simulink model "Two_cars_multi_agent"  (Simulink 8.3)
settings: Solver=ode45  StartTime=0  StopTime=5  FixedStep=0.1  RelTol=1e-3
PreLoadFcn:
  | d1 = density.Data(2:end);
  | d1 = d1(2:end);
  | mean(d1)
libraries: simulink_extras x9, Solver_SF x3, truetime x3
settings Model: Creator=dhall  LastModifiedBy=Ye  SimulationMode=accelerator  ExtModeTrigMode=oneshot  ExtModeArmWhenConnect=off
settings DataIOCC: LimitDataPoints=off  SignalLoggingName=sigsOut
settings OptimizationCC: BooleanDataType=off  LocalBlockOutputs=off  InitFltsAndDblsToZero=on
settings DebuggingCC: ReadBeforeWriteMsg=DisableAll  WriteAfterWriteMsg=DisableAll  WriteAfterReadMsg=DisableAll  SaveWithParameterizedLinksMsg=none  SolverPrmCheckMsg=none  MultiTaskDSMMsg=none  MultiTaskCondExecSysMsg=none  StateNameClashWarn=none
settings HardwareCC: TargetIntDivRoundTo=Zero  TargetEndianess=LittleEndian  TargetHWDeviceType=MATLAB Host  ProdEqTarget=off
settings ModelReferenceCC: UpdateModelReferenceTargets=IfOutOfDate
settings SFSimCC: SFSimEnableDebug=off  SFSimOverflowDetection=off  SFSimEcho=off
settings RTWCC: IncludeERTFirstTime=on
settings GRTTargetCC: TargetFcnLib=ansi_tfl_tmw.mat  CompOptLevelCompliant=off

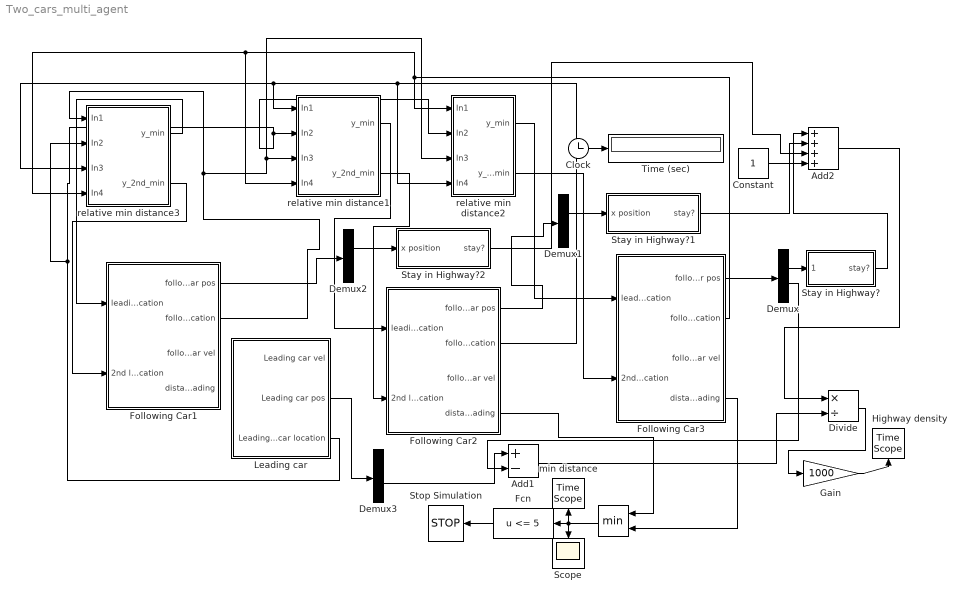
== system Two_cars_multi_agent ==
  " " : MinMax  Inputs=2  SampleTime=0.1
  Add1 : Sum  Inputs=+-
  Add2 : Sum  Inputs=++++
  Clock : Clock
  Constant : Constant
  Demux{,1..3} (4 alike) : Demux
  Divide : Product  Inputs=*/  RndMeth=Ceiling
  Fcn : Fcn  Expr=u <= 5
  "Following Car1 " : Subsystem
  Following Car2 : Subsystem
  Following Car3 : Subsystem
  Gain : Gain  Gain=1000
  Highway density : TimeScope  DefaultConfigurationName=spbscopes.TimeScopeBlockCfg  ScopeSpecification=DataTag1
  Leading car : Subsystem
  Scope : Scope
      settings: YMin=0  YMax=50  SaveName=ScopeData2
  Stay in Highway? : Subsystem
  Stay in Highway?1 : Subsystem
  Stay in Highway?2 : Subsystem
  Stop Simulation : Stop
  Time (sec) : Display
      settings: Format=bank  Decimation=100
  min distance : TimeScope  DefaultConfigurationName=spbscopes.TimeScopeBlockCfg  ScopeSpecification=DataTag2
  relative min distance1 : Subsystem
  relative min distance2 : Subsystem
  relative min distance3 : Subsystem
  wires:
  Clock/1 -> Time (sec)/1
  Fcn/1 -> Stop Simulation/1
  "Following Car1 "/2(following car location) -> relative min distance1/3(In3), relative min distance2/3(In3), relative min distance3/1(In1)
  Leading car/3(Leading car location) -> relative min distance2/2(In2), relative min distance1/2(In2), relative min distance3/2(In2)
  Leading car/2(Leading car pos) -> Demux3/1
  Following Car2/1(following car pos) -> Demux1/1
  Following Car2/2(following car location) -> relative min distance2/4(In4), relative min distance3/3(In3), relative min distance1/1(In1)
  Following Car3/1(following car pos) -> Demux/1
  Following Car3/2(following car location) -> relative min distance3/4(In4), relative min distance1/4(In4), relative min distance2/1(In1)
  relative min distance3/1(y_min) -> "Following Car1 "/1(leading car location)
  relative min distance1/1(y_min) -> Following Car2/1(leading car location)
  relative min distance2/1(y_min) -> Following Car3/1(leading car location)
  Add1/1 -> Divide/2
  Demux/2 -> Stay in Highway?/1(x position)
  Stay in Highway?/1(stay?) -> Add2/1
  Demux1/2 -> Stay in Highway?1/1(x position)
  Stay in Highway?1/1(stay?) -> Add2/2
  Demux2/2 -> Stay in Highway?2/1(x position)
  Stay in Highway?2/1(stay?) -> Add2/3
  Demux3/3 -> Add1/1
  Demux/3 -> Add1/2
  Constant/1 -> Add2/4
  Divide/1 -> Gain/1
  Add2/1 -> Divide/1
  Gain/1 -> Highway density/1
  relative min distance2/2(y_2nd_min) -> Following Car3/2(2nd leading car location)
  "Following Car1 "/1(following car pos) -> Demux2/1
  relative min distance1/2(y_2nd_min) -> Following Car2/2(2nd leading car location)
  relative min distance3/2(y_2nd_min) -> "Following Car1 "/2(2nd leading car location)
  Following Car2/4(distance leading) -> " "/1
  " "/1 -> Scope/1, Fcn/1, min distance/1
  Following Car3/4(distance leading) -> " "/2

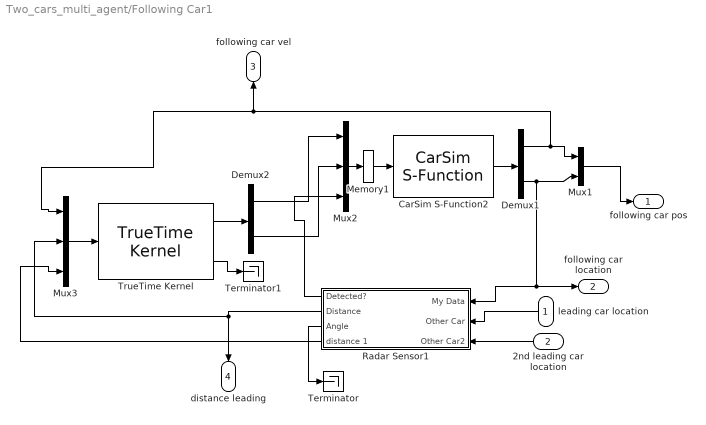
== system Two_cars_multi_agent/Following Car1  ==
  leading car location : Inport
  2nd leading car location : Inport  Port=2
  CarSim S-Function2 : Solver_SF/CarSim S-Function  Priority=1  VehicleCode=i_i2  SIMFILE=following_car_1.sim
  Demux1 : Demux  Outputs=[1 3]
  Demux2 : Demux  Outputs=[1 1]
  Memory1 : Memory
  Mux1 : Mux  Inputs=2
  Mux2 : Mux  Inputs=3
  Mux3 : Mux  Inputs=3
  Radar Sensor1 : Subsystem  mask{S_ANGLE=360, S_DISTANCE=700}
      mask prompts: S_ANGLE "View Angle (deg)"; S_DISTANCE "Distance Range (m)"
      mask help:
      | An example of a radar sensor. It can detect the distance between the sensor and another object according its position (Xo, Yo).
      |
      | Input parameters are View Angle(deg) and radar detectable distance(m).
      mask init:
      | d_ang= str2double(S_ANGLE)/2;
      | set_param([gcb '/View Angle'], 'Threshold', sprintf('%0.2f', d_ang));
      | set_param([gcb '/L-Radar'], 'Value', S_DISTANCE);
  Terminator : Terminator
  Terminator1 : Terminator
  TrueTime Kernel : truetime/TrueTime Kernel  sfun=controller_init_cpp  args=1  ninputsoutputs=[3 2]  ntriggers=0  trigtype=falling  nwnodenbr=[]  clockoffsetdrift=[0 0]  schedoutput=on  battery=off  poweroutput=off
  following car pos : Outport
  following car location : Outport  Port=2
  following car vel : Outport  Port=3
  distance leading : Outport  Port=4
  wires:
  Demux1/2 -> Mux1/2, Radar Sensor1/1(My Data), following car location/1
  CarSim S-Function2/1 -> Demux1/1
  Demux1/1 -> Mux1/1, Mux3/1, following car vel/1
  Memory1/1 -> CarSim S-Function2/1
  Mux2/1 -> Memory1/1
  Radar Sensor1/2(Distance) -> Mux3/2, distance leading/1
  Radar Sensor1/1(Detected?) -> Mux2/3
  Mux1/1 -> following car pos/1
  leading car location/1 -> Radar Sensor1/2(Other Car)
  Demux2/1 -> Mux2/1
  Demux2/2 -> Mux2/2
  2nd leading car location/1 -> Radar Sensor1/3(Other Car2)
  Radar Sensor1/3(Angle) -> Terminator/1
  Radar Sensor1/4(distance 1) -> Mux3/3
  TrueTime Kernel/1 -> Demux2/1
  Mux3/1 -> TrueTime Kernel/1
  TrueTime Kernel/2 -> Terminator1/1

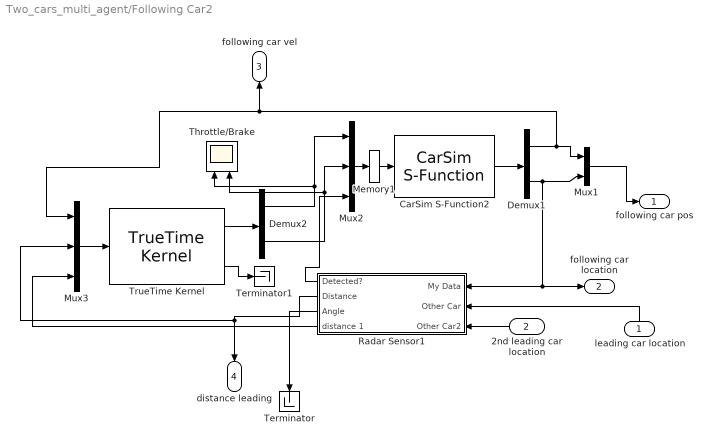
== system Two_cars_multi_agent/Following Car2 ==
  leading car location : Inport
  2nd leading car location : Inport  Port=2
  CarSim S-Function2 : Solver_SF/CarSim S-Function  Priority=1  VehicleCode=i_i2_2  SIMFILE=following_car_2.sim
  Demux1 : Demux  Outputs=[1 3]
  Demux2 : Demux  Outputs=[1 1]
  Memory1 : Memory
  Mux1 : Mux  Inputs=2
  Mux2 : Mux  Inputs=3
  Mux3 : Mux  Inputs=3
  Radar Sensor1 : Subsystem  mask{S_ANGLE=360, S_DISTANCE=700}
      mask prompts: S_ANGLE "View Angle (deg)"; S_DISTANCE "Distance Range (m)"
      mask help:
      | An example of a radar sensor. It can detect the distance between the sensor and another object according its position (Xo, Yo).
      |
      | Input parameters are View Angle(deg) and radar detectable distance(m).
      mask init:
      | d_ang= str2double(S_ANGLE)/2;
      | set_param([gcb '/View Angle'], 'Threshold', sprintf('%0.2f', d_ang));
      | set_param([gcb '/L-Radar'], 'Value', S_DISTANCE);
  Terminator : Terminator
  Terminator1 : Terminator
  Throttle/Brake : Scope  NumInputPorts=2
      settings: TickLabels=on  TimeRange=50  YMin=0~0  YMax=1~12.5  MaxDataPoints=50000  SampleTime=100
  TrueTime Kernel : truetime/TrueTime Kernel  sfun=controller_init_cpp  args=1  ninputsoutputs=[3 2]  ntriggers=0  trigtype=falling  nwnodenbr=[]  clockoffsetdrift=[0 0]  schedoutput=on  battery=off  poweroutput=off
  following car pos : Outport
  following car location : Outport  Port=2
  following car vel : Outport  Port=3
  distance leading : Outport  Port=4
  wires:
  Demux1/2 -> Mux1/2, Radar Sensor1/1(My Data), following car location/1
  Demux1/1 -> Mux1/1, Mux3/1, following car vel/1
  Memory1/1 -> CarSim S-Function2/1
  Mux2/1 -> Memory1/1
  Radar Sensor1/2(Distance) -> Mux3/2, distance leading/1
  Radar Sensor1/1(Detected?) -> Mux2/3
  Mux1/1 -> following car pos/1
  leading car location/1 -> Radar Sensor1/2(Other Car)
  CarSim S-Function2/1 -> Demux1/1
  Demux2/1 -> Mux2/1, Throttle/Brake/1
  Demux2/2 -> Mux2/2, Throttle/Brake/2
  2nd leading car location/1 -> Radar Sensor1/3(Other Car2)
  Radar Sensor1/3(Angle) -> Terminator/1
  Radar Sensor1/4(distance 1) -> Mux3/3
  TrueTime Kernel/1 -> Demux2/1
  Mux3/1 -> TrueTime Kernel/1
  TrueTime Kernel/2 -> Terminator1/1

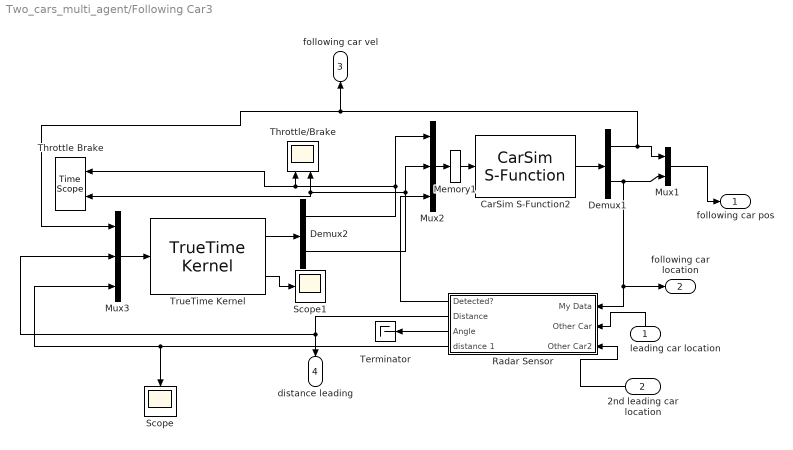
== system Two_cars_multi_agent/Following Car3 ==
  leading car location : Inport
  2nd leading car location : Inport  Port=2
  CarSim S-Function2 : Solver_SF/CarSim S-Function  Priority=1  VehicleCode=i_i2_3  SIMFILE=following_car_3.sim
  Demux1 : Demux  Outputs=[1 3]
  Demux2 : Demux  Outputs=[1 1]
  Memory1 : Memory
  Mux1 : Mux  Inputs=2
  Mux2 : Mux  Inputs=3
  Mux3 : Mux  Inputs=3
  Radar Sensor : Subsystem  mask{S_ANGLE=360, S_DISTANCE=700}
      mask prompts: S_ANGLE "View Angle (deg)"; S_DISTANCE "Distance Range (m)"
      mask help:
      | An example of a radar sensor. It can detect the distance between the sensor and another object according its position (Xo, Yo).
      |
      | Input parameters are View Angle(deg) and radar detectable distance(m).
      mask init:
      | d_ang= str2double(S_ANGLE)/2;
      | set_param([gcb '/View Angle'], 'Threshold', sprintf('%0.2f', d_ang));
      | set_param([gcb '/L-Radar'], 'Value', S_DISTANCE);
  Scope : Scope
      settings: YMin=150  YMax=320
  Scope1 : Scope
      settings: YMin=150  YMax=320  SaveName=ScopeData3
  Terminator : Terminator
  Throttle Brake : TimeScope  NumInputPorts=2  DefaultConfigurationName=spbscopes.TimeScopeBlockCfg  ScopeSpecification=DataTag0
  Throttle/Brake : Scope  NumInputPorts=2
      settings: TickLabels=on  TimeRange=50  YMin=0~0  YMax=1~12.5  MaxDataPoints=50000  SampleTime=100
  TrueTime Kernel : truetime/TrueTime Kernel  sfun=controller_init_cpp  args=1  ninputsoutputs=[3 2]  ntriggers=0  trigtype=falling  nwnodenbr=[]  clockoffsetdrift=[0 0]  schedoutput=on  battery=off  poweroutput=off
  following car pos : Outport
  following car location : Outport  Port=2
  following car vel : Outport  Port=3
  distance leading : Outport  Port=4
  wires:
  Demux1/2 -> Mux1/2, following car location/1, Radar Sensor/1(My Data)
  CarSim S-Function2/1 -> Demux1/1
  Demux1/1 -> Mux1/1, Mux3/1, following car vel/1
  Memory1/1 -> CarSim S-Function2/1
  Mux2/1 -> Memory1/1
  Radar Sensor/2(Distance) -> Mux3/2, distance leading/1
  Radar Sensor/1(Detected?) -> Mux2/3
  Mux1/1 -> following car pos/1
  leading car location/1 -> Radar Sensor/2(Other Car)
  Demux2/1 -> Mux2/1, Throttle Brake/1, Throttle/Brake/1
  Demux2/2 -> Mux2/2, Throttle/Brake/2, Throttle Brake/2
  Radar Sensor/3(Angle) -> Terminator/1
  Radar Sensor/4(distance 1) -> Mux3/3, Scope/1
  2nd leading car location/1 -> Radar Sensor/3(Other Car2)
  TrueTime Kernel/1 -> Demux2/1
  Mux3/1 -> TrueTime Kernel/1
  TrueTime Kernel/2 -> Scope1/1

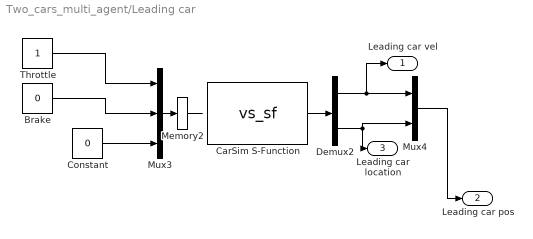
== system Two_cars_multi_agent/Leading car ==
  Brake : Constant  Value=0
  CarSim S-Function : S-Function  Priority=1  AncestorBlock=Solver_SF/CarSim S-Function  FunctionName=vs_sf  Parameters='Leading_car.sim'  EnableBusSupport=off  mask(Vehicle math model library){VehicleCode=i_i, SIMFILE=Leading_car.sim}
      mask prompts: VehicleCode "Vehicle code (for instance i_i, i_s, i_i__ss):"; SIMFILE "Simfile name:"
      mask help:
      | The vehicle code on this S-Function determine which solver is used for vehicle type that is simulated.
      |
      | Simfile lists the names of the main files that will be read and written by the solver program.
      mask init:
      | set_param(gcb, 'Parameters', ['''',SIMFILE,'''']);
      settings: AttributesFormatString=Vehicle Code: %<VehicleCode>
      mask Display: image(imread('car_simulink.bmp'))
  Constant : Constant  Value=0
  Demux2 : Demux  Outputs=[1 3]
  Memory2 : Memory
  Mux3 : Mux  Inputs=3
  Mux4 : Mux  Inputs=2
  Throttle : Constant
  Leading car vel : Outport
  Leading car pos : Outport  Port=2
  Leading car location : Outport  Port=3
  wires:
  Throttle/1 -> Mux3/1
  CarSim S-Function/1 -> Demux2/1
  Mux3/1 -> Memory2/1
  Constant/1 -> Mux3/3
  Brake/1 -> Mux3/2
  Demux2/2 -> Leading car location/1, Mux4/2
  Mux4/1 -> Leading car pos/1
  Demux2/1 -> Leading car vel/1, Mux4/1
  Memory2/1 -> ?

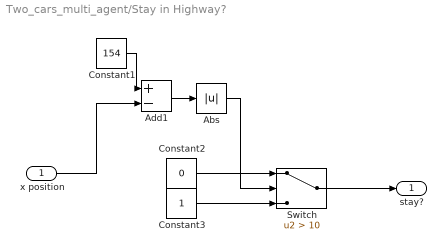
== system Two_cars_multi_agent/Stay in Highway? ==
  x position : Inport
  Abs : Abs
  Add1 : Sum  Inputs=+-
  Constant1 : Constant  Value=154
  Constant2 : Constant  Value=0
  Constant3 : Constant
  Switch : Switch  Criteria=u2 > Threshold  Threshold=10
  stay? : Outport
  wires:
  Constant3/1 -> Switch/3
  x position/1 -> Add1/2
  Constant2/1 -> Switch/1
  Switch/1 -> stay?/1
  Constant1/1 -> Add1/1
  Add1/1 -> Abs/1
  Abs/1 -> Switch/2

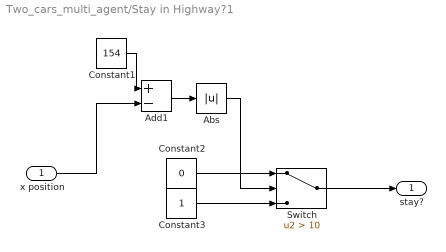
== system Two_cars_multi_agent/Stay in Highway?1 ==
  x position : Inport
  Abs : Abs
  Add1 : Sum  Inputs=+-
  Constant1 : Constant  Value=154
  Constant2 : Constant  Value=0
  Constant3 : Constant
  Switch : Switch  Criteria=u2 > Threshold  Threshold=10
  stay? : Outport
  wires:
  Abs/1 -> Switch/2
  Add1/1 -> Abs/1
  Constant1/1 -> Add1/1
  Switch/1 -> stay?/1
  Constant2/1 -> Switch/1
  x position/1 -> Add1/2
  Constant3/1 -> Switch/3

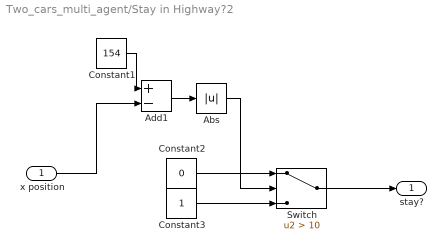
== system Two_cars_multi_agent/Stay in Highway?2 ==
  x position : Inport
  Abs : Abs
  Add1 : Sum  Inputs=+-
  Constant1 : Constant  Value=154
  Constant2 : Constant  Value=0
  Constant3 : Constant
  Switch : Switch  Criteria=u2 > Threshold  Threshold=10
  stay? : Outport
  wires:
  Constant3/1 -> Switch/3
  x position/1 -> Add1/2
  Constant2/1 -> Switch/1
  Switch/1 -> stay?/1
  Constant1/1 -> Add1/1
  Add1/1 -> Abs/1
  Abs/1 -> Switch/2

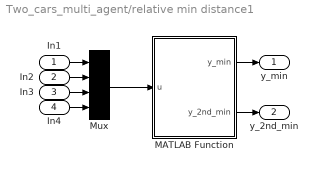
== system Two_cars_multi_agent/relative min distance1 ==
  In1 : Inport
  In2 : Inport  Port=2
  In3 : Inport  Port=3
  In4 : Inport  Port=4
  MATLAB Function : MATLAB Function  TreatAsAtomicUnit=on
  Mux : Mux
  y_min : Outport
  y_2nd_min : Outport  Port=2
  wires:
  Mux/1 -> MATLAB Function/1(u)
  In2/1 -> Mux/2
  In4/1 -> Mux/4
  In1/1 -> Mux/1
  MATLAB Function/1(y_min) -> y_min/1
  In3/1 -> Mux/3
  MATLAB Function/2(y_2nd_min) -> y_2nd_min/1

== system Two_cars_multi_agent/relative min distance2 ==
  In1 : Inport
  In2 : Inport  Port=2
  In3 : Inport  Port=3
  In4 : Inport  Port=4
  MATLAB Function : MATLAB Function  TreatAsAtomicUnit=on
  Mux : Mux
  y_min : Outport
  y_2nd_min : Outport  Port=2
  wires:
  Mux/1 -> MATLAB Function/1(u)
  In2/1 -> Mux/2
  In4/1 -> Mux/4
  In1/1 -> Mux/1
  MATLAB Function/1(y_min) -> y_min/1
  In3/1 -> Mux/3
  MATLAB Function/2(y_2nd_min) -> y_2nd_min/1

== system Two_cars_multi_agent/relative min distance3 ==
  In1 : Inport
  In2 : Inport  Port=2
  In3 : Inport  Port=3
  In4 : Inport  Port=4
  MATLAB Function : MATLAB Function  TreatAsAtomicUnit=on
  Mux : Mux
  y_min : Outport
  y_2nd_min : Outport  Port=2
  wires:
  Mux/1 -> MATLAB Function/1(u)
  In2/1 -> Mux/2
  In4/1 -> Mux/4
  In1/1 -> Mux/1
  MATLAB Function/1(y_min) -> y_min/1
  In3/1 -> Mux/3
  MATLAB Function/2(y_2nd_min) -> y_2nd_min/1

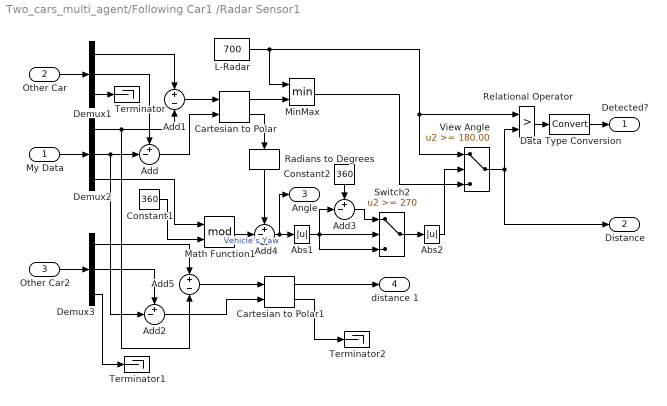
== system Two_cars_multi_agent/Following Car1 /Radar Sensor1 ==
  My Data : Inport
  Other Car : Inport  Port=2
  Other Car2 : Inport  Port=3
  Abs1 : Abs
  Abs2 : Abs
  Add{,2..4} (4 alike) : Sum  Inputs=+-|
  Add1 : Sum  Inputs=+-
  Add5 : Sum  Inputs=+-
  Cartesian to Polar : simulink_extras/Transformations/Cartesian to Polar
  Cartesian to Polar1 : simulink_extras/Transformations/Cartesian to Polar
  Constant1 : Constant  Value=360
  Constant2 : Constant  Value=360
  Data Type Conversion : DataTypeConversion  RndMeth=Zero
  Demux1 : Demux  Outputs=3
  Demux2 : Demux  Outputs=3
  Demux3 : Demux  Outputs=3
  L-Radar : Constant  Value=700
  Math Function1 : Math  Operator=mod  SaturateOnIntegerOverflow=on
  MinMax : MinMax  Inputs=2  SaturateOnIntegerOverflow=on  InputSameDT=on
  Radians to Degrees : simulink_extras/Transformations/Radians to Degrees
  Relational Operator : RelationalOperator  Operator=>  OutDataTypeStr=boolean
  Switch2 : Switch  Threshold=270
  Terminator : Terminator
  Terminator1 : Terminator
  Terminator2 : Terminator
  View Angle : Switch  Threshold=180.00
  Detected? : Outport
  Distance : Outport  Port=2
  Angle : Outport  Port=3
  distance 1 : Outport  Port=4
  wires:
  Demux2/3 -> Math Function1/1
  Constant1/1 -> Math Function1/2
  Add/1 -> Cartesian to Polar/2
  Add1/1 -> Cartesian to Polar/1
  Demux2/1 -> Add5/2, Add1/2
  Demux1/1 -> Add1/1
  Demux2/2 -> Add2/2, Add/2
  Demux1/2 -> Add/1
  Demux1/3 -> Terminator/1
  My Data/1 -> Demux2/1
  Other Car/1 -> Demux1/1
  Math Function1/1 -> Add4/2  "Vehicle's Yaw"
  Add4/1 -> Angle/1, Abs1/1
  Abs1/1 -> Switch2/2, Add3/2, Switch2/3
  Add3/1 -> Switch2/1
  Constant2/1 -> Add3/1
  L-Radar/1 -> MinMax/1, View Angle/1, Relational Operator/1
  MinMax/1 -> View Angle/3
  Switch2/1 -> Abs2/1
  Abs2/1 -> View Angle/2
  View Angle/1 -> Distance/1, Relational Operator/2
  Relational Operator/1 -> Data Type Conversion/1
  Data Type Conversion/1 -> Detected?/1
  Radians to Degrees/1 -> Add4/1
  Cartesian to Polar/1 -> MinMax/2
  Cartesian to Polar/2 -> Radians to Degrees/1
  Other Car2/1 -> Demux3/1
  Demux3/1 -> Add5/1
  Demux3/2 -> Add2/1
  Demux3/3 -> Terminator1/1
  Add5/1 -> Cartesian to Polar1/1
  Add2/1 -> Cartesian to Polar1/2
  Cartesian to Polar1/1 -> distance 1/1
  Cartesian to Polar1/2 -> Terminator2/1

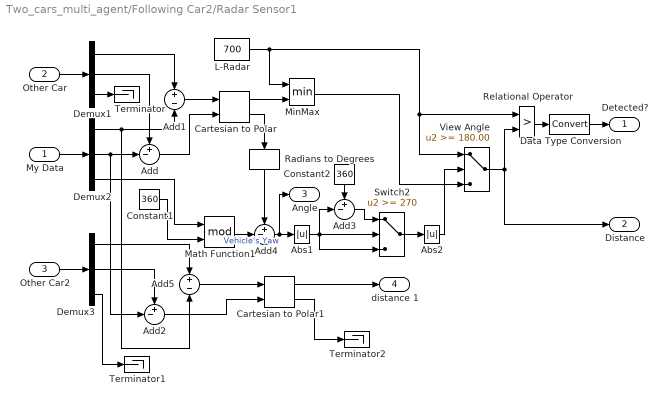
== system Two_cars_multi_agent/Following Car2/Radar Sensor1 ==
  My Data : Inport
  Other Car : Inport  Port=2
  Other Car2 : Inport  Port=3
  Abs1 : Abs
  Abs2 : Abs
  Add{,2..4} (4 alike) : Sum  Inputs=+-|
  Add1 : Sum  Inputs=+-
  Add5 : Sum  Inputs=+-
  Cartesian to Polar : simulink_extras/Transformations/Cartesian to Polar
  Cartesian to Polar1 : simulink_extras/Transformations/Cartesian to Polar
  Constant1 : Constant  Value=360
  Constant2 : Constant  Value=360
  Data Type Conversion : DataTypeConversion  RndMeth=Zero
  Demux1 : Demux  Outputs=3
  Demux2 : Demux  Outputs=3
  Demux3 : Demux  Outputs=3
  L-Radar : Constant  Value=700
  Math Function1 : Math  Operator=mod  SaturateOnIntegerOverflow=on
  MinMax : MinMax  Inputs=2  SaturateOnIntegerOverflow=on  InputSameDT=on
  Radians to Degrees : simulink_extras/Transformations/Radians to Degrees
  Relational Operator : RelationalOperator  Operator=>  OutDataTypeStr=boolean
  Switch2 : Switch  Threshold=270
  Terminator : Terminator
  Terminator1 : Terminator
  Terminator2 : Terminator
  View Angle : Switch  Threshold=180.00
  Detected? : Outport
  Distance : Outport  Port=2
  Angle : Outport  Port=3
  distance 1 : Outport  Port=4
  wires:
  Demux2/3 -> Math Function1/1
  Constant1/1 -> Math Function1/2
  Add/1 -> Cartesian to Polar/2
  Add1/1 -> Cartesian to Polar/1
  Demux2/1 -> Add5/2, Add1/2
  Demux1/1 -> Add1/1
  Demux2/2 -> Add2/2, Add/2
  Demux1/2 -> Add/1
  Demux1/3 -> Terminator/1
  My Data/1 -> Demux2/1
  Other Car/1 -> Demux1/1
  Math Function1/1 -> Add4/2  "Vehicle's Yaw"
  Add4/1 -> Angle/1, Abs1/1
  Abs1/1 -> Switch2/2, Add3/2, Switch2/3
  Add3/1 -> Switch2/1
  Constant2/1 -> Add3/1
  L-Radar/1 -> MinMax/1, View Angle/1, Relational Operator/1
  MinMax/1 -> View Angle/3
  Switch2/1 -> Abs2/1
  Abs2/1 -> View Angle/2
  View Angle/1 -> Distance/1, Relational Operator/2
  Relational Operator/1 -> Data Type Conversion/1
  Data Type Conversion/1 -> Detected?/1
  Radians to Degrees/1 -> Add4/1
  Cartesian to Polar/1 -> MinMax/2
  Cartesian to Polar/2 -> Radians to Degrees/1
  Other Car2/1 -> Demux3/1
  Demux3/1 -> Add5/1
  Demux3/2 -> Add2/1
  Demux3/3 -> Terminator1/1
  Add5/1 -> Cartesian to Polar1/1
  Add2/1 -> Cartesian to Polar1/2
  Cartesian to Polar1/1 -> distance 1/1
  Cartesian to Polar1/2 -> Terminator2/1

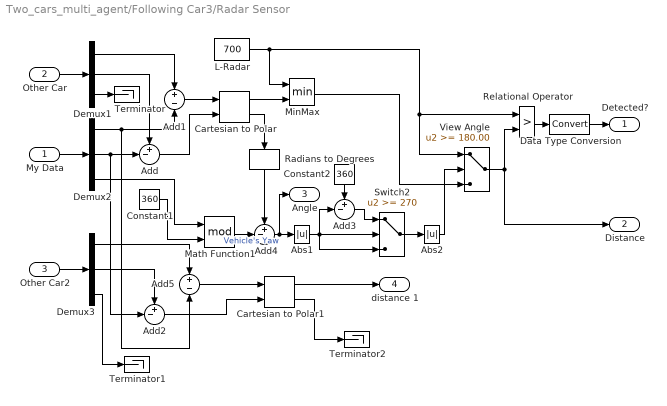
== system Two_cars_multi_agent/Following Car3/Radar Sensor ==
  My Data : Inport
  Other Car : Inport  Port=2
  Other Car2 : Inport  Port=3
  Abs1 : Abs
  Abs2 : Abs
  Add{,2..4} (4 alike) : Sum  Inputs=+-|
  Add1 : Sum  Inputs=+-
  Add5 : Sum  Inputs=+-
  Cartesian to Polar : simulink_extras/Transformations/Cartesian to Polar
  Cartesian to Polar1 : simulink_extras/Transformations/Cartesian to Polar
  Constant1 : Constant  Value=360
  Constant2 : Constant  Value=360
  Data Type Conversion : DataTypeConversion  RndMeth=Zero
  Demux1 : Demux  Outputs=3
  Demux2 : Demux  Outputs=3
  Demux3 : Demux  Outputs=3
  L-Radar : Constant  Value=700
  Math Function1 : Math  Operator=mod  SaturateOnIntegerOverflow=on
  MinMax : MinMax  Inputs=2  SaturateOnIntegerOverflow=on  InputSameDT=on
  Radians to Degrees : simulink_extras/Transformations/Radians to Degrees
  Relational Operator : RelationalOperator  Operator=>  OutDataTypeStr=boolean
  Switch2 : Switch  Threshold=270
  Terminator : Terminator
  Terminator1 : Terminator
  Terminator2 : Terminator
  View Angle : Switch  Threshold=180.00
  Detected? : Outport
  Distance : Outport  Port=2
  Angle : Outport  Port=3
  distance 1 : Outport  Port=4
  wires:
  Demux2/3 -> Math Function1/1
  Constant1/1 -> Math Function1/2
  Add/1 -> Cartesian to Polar/2
  Add1/1 -> Cartesian to Polar/1
  Demux2/1 -> Add5/2, Add1/2
  Demux1/1 -> Add1/1
  Demux2/2 -> Add2/2, Add/2
  Demux1/2 -> Add/1
  Demux1/3 -> Terminator/1
  My Data/1 -> Demux2/1
  Other Car/1 -> Demux1/1
  Math Function1/1 -> Add4/2  "Vehicle's Yaw"
  Add4/1 -> Angle/1, Abs1/1
  Abs1/1 -> Switch2/2, Add3/2, Switch2/3
  Add3/1 -> Switch2/1
  Constant2/1 -> Add3/1
  L-Radar/1 -> MinMax/1, View Angle/1, Relational Operator/1
  MinMax/1 -> View Angle/3
  Switch2/1 -> Abs2/1
  Abs2/1 -> View Angle/2
  View Angle/1 -> Distance/1, Relational Operator/2
  Relational Operator/1 -> Data Type Conversion/1
  Data Type Conversion/1 -> Detected?/1
  Radians to Degrees/1 -> Add4/1
  Cartesian to Polar/1 -> MinMax/2
  Cartesian to Polar/2 -> Radians to Degrees/1
  Other Car2/1 -> Demux3/1
  Demux3/1 -> Add5/1
  Demux3/2 -> Add2/1
  Demux3/3 -> Terminator1/1
  Add5/1 -> Cartesian to Polar1/1
  Add2/1 -> Cartesian to Polar1/2
  Cartesian to Polar1/1 -> distance 1/1
  Cartesian to Polar1/2 -> Terminator2/1

== matlab function relative min distance1/MATLAB Function ==
  data: u input double; y_min output double; y_2nd_min output double
function [y_min, y_2nd_min]  = fcn(u)
%#codegen
me = u(1:3);
car1 = u(4:6);
car2 = u(7:9);
car3 = u(10:12);
candidates = [car1';car2';car3'];

distance_y = [car1(2) - me(2), car2(2) - me(2), car3(2) - me(2)];
distance_y(distance_y < 0) = inf;
distance_x = [car1(1) - me(1), car2(1) - me(1), car3(1) - me(1)];
distance = sqrt((distance_x .^ 2 + distance_y .^ 2));
% distance = [car1(2) - me(2), car2(2) - me(2), car3(2) - me(2)];
% distance(distance < 0) = inf;
[v_min, i_min] = min(distance);
distance(i_min) = inf;
[v_2nd_min, i_2nd_min] = min(distance);


% if i == 1
%     y = car1;
% elseif i == 2
%     y = car2;
% else
%     y = car3;
% end

y_min = candidates(i_min, :)';
y_2nd_min = candidates(i_2nd_min, :)';

% y = car2;
% 
% function y = fcn(u)
% %#codegen
% me = u(1:3);
% car1 = u(4:6);
% car2 = u(7:9);
% car3 = u(10:12);
% candidates = [car1';car2';car3'];
% 
% distance_y = [car1(2) - me(2), car2(2) - me(2), car3(2) - me(2)];
% distance_y(distance_y < 0) = inf;
% distance_x = [car1(1) - me(1), car2(1) - me(1), car3(1) - me(1)];
% distance = sqrt((distance_x .^ 2 + distance_y .^ 2));
% % distance = [car1(2) - me(2), car2(2) - me(2), car3(2) - me(2)];
% % distance(distance < 0) = inf;
% [v, i] = min(distance);
% 
% % if i == 1
% %     y = car1;
% % elseif i == 2
% %     y = car2;
% % else
% %     y = car3;
% % end
% 
% y = candidates(i, :)';
% 
% % y = car2;

== matlab function relative min distance3/MATLAB Function ==
  data: u input double; y_min output double; y_2nd_min output double
function [y_min, y_2nd_min]  = fcn(u)
%#codegen
me = u(1:3);
car1 = u(4:6);
car2 = u(7:9);
car3 = u(10:12);
candidates = [car1';car2';car3'];

distance_y = [car1(2) - me(2), car2(2) - me(2), car3(2) - me(2)];
distance_y(distance_y < 0) = inf;
distance_x = [car1(1) - me(1), car2(1) - me(1), car3(1) - me(1)];
distance = sqrt((distance_x .^ 2 + distance_y .^ 2));
% distance = [car1(2) - me(2), car2(2) - me(2), car3(2) - me(2)];
% distance(distance < 0) = inf;
[v_min, i_min] = min(distance);
distance(i_min) = inf;
[v_2nd_min, i_2nd_min] = min(distance);


% if i == 1
%     y = car1;
% elseif i == 2
%     y = car2;
% else
%     y = car3;
% end

y_min = candidates(i_min, :)';
y_2nd_min = candidates(i_2nd_min, :)';

% y = car2;
% 
% function y = fcn(u)
% %#codegen
% me = u(1:3);
% car1 = u(4:6);
% car2 = u(7:9);
% car3 = u(10:12);
% candidates = [car1';car2';car3'];
% 
% distance_y = [car1(2) - me(2), car2(2) - me(2), car3(2) - me(2)];
% distance_y(distance_y < 0) = inf;
% distance_x = [car1(1) - me(1), car2(1) - me(1), car3(1) - me(1)];
% distance = sqrt((distance_x .^ 2 + distance_y .^ 2));
% % distance = [car1(2) - me(2), car2(2) - me(2), car3(2) - me(2)];
% % distance(distance < 0) = inf;
% [v, i] = min(distance);
% 
% % if i == 1
% %     y = car1;
% % elseif i == 2
% %     y = car2;
% % else
% %     y = car3;
% % end
% 
% y = candidates(i, :)';
% 
% % y = car2;

== matlab function relative min distance2/MATLAB Function ==
  data: u input double; y_min output double; y_2nd_min output double
function [y_min, y_2nd_min]  = fcn(u)
%#codegen
me = u(1:3);
car1 = u(4:6);
car2 = u(7:9);
car3 = u(10:12);
candidates = [car1';car2';car3'];

distance_y = [car1(2) - me(2), car2(2) - me(2), car3(2) - me(2)];
distance_y(distance_y < 0) = inf;
distance_x = [car1(1) - me(1), car2(1) - me(1), car3(1) - me(1)];
distance = sqrt((distance_x .^ 2 + distance_y .^ 2));
% distance = [car1(2) - me(2), car2(2) - me(2), car3(2) - me(2)];
% distance(distance < 0) = inf;
[v_min, i_min] = min(distance);
distance(i_min) = inf;
[v_2nd_min, i_2nd_min] = min(distance);


% if i == 1
%     y = car1;
% elseif i == 2
%     y = car2;
% else
%     y = car3;
% end

y_min = candidates(i_min, :)';
y_2nd_min = candidates(i_2nd_min, :)';

% y = car2;
% 
% function y = fcn(u)
% %#codegen
% me = u(1:3);
% car1 = u(4:6);
% car2 = u(7:9);
% car3 = u(10:12);
% candidates = [car1';car2';car3'];
% 
% distance_y = [car1(2) - me(2), car2(2) - me(2), car3(2) - me(2)];
% distance_y(distance_y < 0) = inf;
% distance_x = [car1(1) - me(1), car2(1) - me(1), car3(1) - me(1)];
% distance = sqrt((distance_x .^ 2 + distance_y .^ 2));
% % distance = [car1(2) - me(2), car2(2) - me(2), car3(2) - me(2)];
% % distance(distance < 0) = inf;
% [v, i] = min(distance);
% 
% % if i == 1
% %     y = car1;
% % elseif i == 2
% %     y = car2;
% % else
% %     y = car3;
% % end
% 
% y = candidates(i, :)';
% 
% % y = car2;
